simulink model "mbdt_autosar_system_top"  (R2019a)
settings: Solver=ode4  StartTime=0  StopTime=1.5  FixedStep=0.005  RelTol=1e-3  EnableMultiTasking=on
InitFcn:
  | mbd_s32k_as_consistency_checks(bdroot(gcs));
model workspace (MAT data in the model file):
  HBridgeCmd_LkupTbl = Simulink.LookupTable
  HBridgeCmd_LkupTbl.Table = Simulink.lookuptable.Table
  HBridgeCmd_LkupTbl.Table.Value = [-2048 -1843 -1638 -1434 -1229 -1024 -819 -614 -410 -205 0 205 410 614 819 1024 1229 1434 1638 1843 2048]
  HBridgeCmd_LkupTbl.Table.Dimensions = [1 21]
  HBridgeCmd_LkupTbl.Table.DataType = 'int16'
  HBridgeCmd_LkupTbl.Table.FieldName = 'Table'
  HBridgeCmd_LkupTbl.Breakpoints = Simulink.lookuptable.Breakpoint
  HBridgeCmd_LkupTbl.Breakpoints.Value = [-100 -90 -80 -70 -60 -50 -40 -30 -20 -10 0 10 20 30 40 50 60 70 80 90 100]
  HBridgeCmd_LkupTbl.Breakpoints.TunableSizeName = 'N1'
  HBridgeCmd_LkupTbl.Breakpoints.Dimensions = [1 21]
  HBridgeCmd_LkupTbl.Breakpoints.DataType = 'single'
  HBridgeCmd_LkupTbl.Breakpoints.FieldName = 'BP1'
  HBridgeCmd_LkupTbl.SupportTunableSize = 0
  HBridgeCmd_LkupTbl.StructTypeInfo = Simulink.lookuptable.StructTypeInfo
  HBridgeCmd_LkupTbl.StructTypeInfo.Name = 'MyStruct_Actuator'
  HBridgeCmd_LkupTbl.StructTypeInfo.DataScope = 'Auto'
  J = 0.226199211484
  Kt = 174.53
  SetpointPercent_LkupTbl = Simulink.LookupTable
  SetpointPercent_LkupTbl.Table = Simulink.lookuptable.Table
  SetpointPercent_LkupTbl.Table.Value = [0 10 20 30 40 50 60 70 80 90 100]
  SetpointPercent_LkupTbl.Table.Dimensions = [1 11]
  SetpointPercent_LkupTbl.Table.DataType = 'single'
  SetpointPercent_LkupTbl.Table.FieldName = 'Table'
  SetpointPercent_LkupTbl.Breakpoints = Simulink.lookuptable.Breakpoint
  SetpointPercent_LkupTbl.Breakpoints.Value = [170 251.5 333 414.5 496 577.5 659 740.5 822 903.5 985]
  SetpointPercent_LkupTbl.Breakpoints.TunableSizeName = 'N1'
  SetpointPercent_LkupTbl.Breakpoints.Dimensions = [1 11]
  SetpointPercent_LkupTbl.Breakpoints.DataType = 'single'
  SetpointPercent_LkupTbl.Breakpoints.FieldName = 'BP1'
  SetpointPercent_LkupTbl.SupportTunableSize = 0
  SetpointPercent_LkupTbl.StructTypeInfo = Simulink.lookuptable.StructTypeInfo
  SetpointPercent_LkupTbl.StructTypeInfo.Name = 'MyStruct'
  SetpointPercent_LkupTbl.StructTypeInfo.DataScope = 'Auto'
  TPSPrimaryPercent_LkupTbl = Simulink.LookupTable
  TPSPrimaryPercent_LkupTbl.Table = Simulink.lookuptable.Table
  TPSPrimaryPercent_LkupTbl.Table.Value = [0 10 20 30 40 50 60 70 80 90 100]
  TPSPrimaryPercent_LkupTbl.Table.Dimensions = [1 11]
  TPSPrimaryPercent_LkupTbl.Table.DataType = 'single'
  TPSPrimaryPercent_LkupTbl.Table.FieldName = 'Table'
  TPSPrimaryPercent_LkupTbl.Breakpoints = Simulink.lookuptable.Breakpoint
  TPSPrimaryPercent_LkupTbl.Breakpoints.Value = [170 249.600006104 329.200012207 408.799987793 488.399993896 568 647.599975586 727.200012207 806.799987793 886.400024414 966]
  TPSPrimaryPercent_LkupTbl.Breakpoints.TunableSizeName = 'N1'
  TPSPrimaryPercent_LkupTbl.Breakpoints.Dimensions = [1 11]
  TPSPrimaryPercent_LkupTbl.Breakpoints.DataType = 'single'
  TPSPrimaryPercent_LkupTbl.Breakpoints.FieldName = 'BP1'
  TPSPrimaryPercent_LkupTbl.SupportTunableSize = 0
  TPSPrimaryPercent_LkupTbl.StructTypeInfo = Simulink.lookuptable.StructTypeInfo
  TPSPrimaryPercent_LkupTbl.StructTypeInfo.Name = 'MyStruct'
  TPSPrimaryPercent_LkupTbl.StructTypeInfo.DataScope = 'Auto'
  TPSSecondaryPercent_LkupTbl = Simulink.LookupTable
  TPSSecondaryPercent_LkupTbl.Table = Simulink.lookuptable.Table
  TPSSecondaryPercent_LkupTbl.Table.Value = [100 90 80 70 60 50 40 30 20 10 0]
  TPSSecondaryPercent_LkupTbl.Table.Dimensions = [1 11]
  TPSSecondaryPercent_LkupTbl.Table.DataType = 'single'
  TPSSecondaryPercent_LkupTbl.Table.FieldName = 'Table'
  TPSSecondaryPercent_LkupTbl.Breakpoints = Simulink.lookuptable.Breakpoint
  TPSSecondaryPercent_LkupTbl.Breakpoints.Value = [170 249.600006104 329.200012207 408.799987793 488.399993896 568 647.599975586 727.200012207 806.799987793 886.400024414 966]
  TPSSecondaryPercent_LkupTbl.Breakpoints.TunableSizeName = 'N1'
  TPSSecondaryPercent_LkupTbl.Breakpoints.Dimensions = [1 11]
  TPSSecondaryPercent_LkupTbl.Breakpoints.DataType = 'single'
  TPSSecondaryPercent_LkupTbl.Breakpoints.FieldName = 'BP1'
  TPSSecondaryPercent_LkupTbl.SupportTunableSize = 0
  TPSSecondaryPercent_LkupTbl.StructTypeInfo = Simulink.lookuptable.StructTypeInfo
  TPSSecondaryPercent_LkupTbl.StructTypeInfo.Name = 'MyStruct'
  TPSSecondaryPercent_LkupTbl.StructTypeInfo.DataScope = 'Auto'
  Ts_verif = Simulink.Parameter
  Ts_verif.Value = 0.001
  Ts_verif.DataType = 'auto'
  Ts_verif.Dimensions = [1 1]
  angle_init = 15
  angle_open = 85
  c = 8.89069171842
  dirtyFlag = 'off'
  fall_end_angle = Simulink.Parameter
  fall_end_angle.Value = 0.1
  fall_end_angle.DataType = 'auto'
  fall_end_angle.Dimensions = [1 1]
  fall_start_angle = Simulink.Parameter
  fall_start_angle.Value = 0.9
  fall_start_angle.DataType = 'auto'
  fall_start_angle.Dimensions = [1 1]
  input_delay = 0.00986306560803
  k = 19.1559540807
  rise_end_angle = Simulink.Parameter
  rise_end_angle.Value = 0.9
  rise_end_angle.DataType = 'auto'
  rise_end_angle.Dimensions = [1 1]
  rise_start_angle = Simulink.Parameter
  rise_start_angle.Value = 0.1
  rise_start_angle.DataType = 'auto'
  rise_start_angle.Dimensions = [1 1]
  vv_fall_time_max = Simulink.Parameter
  vv_fall_time_max.Value = 0.3
  vv_fall_time_max.DataType = 'auto'
  vv_fall_time_max.Dimensions = [1 1]
  vv_fall_time_min = Simulink.Parameter
  vv_fall_time_min.Value = 0.001
  vv_fall_time_min.DataType = 'auto'
  vv_fall_time_min.Dimensions = [1 1]
  vv_rise_time_max = Simulink.Parameter
  vv_rise_time_max.Value = 0.1
  vv_rise_time_max.DataType = 'auto'
  vv_rise_time_max.Dimensions = [1 1]
  vv_rise_time_min = Simulink.Parameter
  vv_rise_time_min.Value = 0.001
  vv_rise_time_min.DataType = 'auto'
  vv_rise_time_min.Dimensions = [1 1]
undefined symbols (not defined in the file or in its folder): sigbuilder_block
libraries: simulink x1
Description:
  | This model shows how to run a throttle position control system AUTOSAR simulation in PIL mode on S32K targets.
  | The model is based on the Matlab's AUTOSAR Blockset Toolbox  'autosar_composition' example. The initial model is a composition containing six interconnected AUTOSAR software components.
  | More details about it can be found here https://www.mathworks.com/help/autosar/ug/example-design-autosar-components.html.
  | 
  | In order to run the entire simulation on S32K target in PIL mode, all the model components were unified in the mbdt_autosar_system.slx model. This was refferenced in the mbdt_autosar_system_top.slx model and
  | the mbdt_autosar_system will be run on target.
  | 
  | In order to run this model in PIL simulation on target, the following steps must be followed:
  | 1. Open the reference 'mbdt_autosar_system' model.
  | 2. Open the 'MBD_S32K1xx_AUTOSAR_Config_Information' block. If you want to run a custom/another AUTOSAR compliant model in PIL, once it runs in simulation as expected, this block must be added in the model.
  | It will change the System target file and will perform the model settings for code build and target deployment.
  | 3. In the MCU Tab chose the processor on which you want to run the model. For S32K11x EVB, the Clock and XTAL Frequency must be 40 MHz/External 40MHz. For the other boards the frequencies must be chosen
  | 80/External 8 MHz.
  | 4. In Build Toolchain Tab select the Compiler which you want to use.
  | 5. In Target Connection Tab Select the Download Interface type: Serial/OpenSDA. The Serial Group selects the computer COM port on which the Matlab model will exchange data with the target and the desired Baud Rate.
  | The OpenSDA group will be active only if the Download Interface is OpenSDA. Here, the right EVB Drive Name must be selected.
  | The PIL Settings Tab selects the EVB board LPUART instance and pins used for the PIL Serial communication. For the S32K11x must be selected the LPUART0/PTB0/PTB1 configuration. For the S32K14x must be selected
  | the LPUART1/PTC6/PTC7 configuration.
  | 6. Save the model and return to the top model.
  | 7. If the top model was never been run on the S32K board, go tho Tools>NXP Model-Based Design AUTOSAR Toolbox for  S32K1xx MCUs>To PIL Mode on S32K.
  | 8. Press Run button.
  | The code will be generated, compiledd, deployed and run on the target.
settings Model: OrderedModelArguments=off  Creator=NXP MBDT Team  LastModifiedBy=nxf35401
settings DataIOCC: SaveFormat=Array  SaveOutput=off  SaveTime=off  ReturnWorkspaceOutputs=off  SignalLoggingName=DataLog
settings OptimizationCC: BooleanDataType=off  DefaultParameterBehavior=Inlined  InlineInvariantSignals=on  EnhancedBackFolding=on  PassReuseOutputArgsAs=Individual arguments  ExpressionDepthLimit=2147483647  ZeroExternalMemoryAtStartup=off  ZeroInternalMemoryAtStartup=off  InitFltsAndDblsToZero=on  NoFixptDivByZeroProtection=on  EfficientFloat2IntCast=on  BufferReusableBoundary=off  OptimizeBlockOrder=speed  DifferentSizesBufferReuse=on
settings DebuggingCC: SaveWithParameterizedLinksMsg=none  MultiTaskDSMMsg=warning  IntegerOverflowMsg=none  ParameterTunabilityLossMsg=error  FcnCallInpInsideContextMsg=warning  BusObjectLabelMismatch=none  StateNameClashWarn=warning  SFUnexpectedBacktrackingDiag=warning  SFNoUnconditionalDefaultTransitionDiag=warning  SFExecutionAtInitializationDiag=none  ArithmeticOperatorsInVariantConditions=warning
settings HardwareCC: ProdBitPerPointer=32  ProdBitPerSizeT=32  ProdBitPerPtrDiffT=32  ProdLargestAtomicInteger=Long  ProdLargestAtomicFloat=Double  ProdWordSize=32  ProdHWDeviceType=ARM Compatible->ARM Cortex
settings ModelReferenceCC: PropagateSignalLabelsOutOfModel=off
settings SFSimCC: SimUseLocalCustomCode=off  SimParseCustomCode=off  MATLABDynamicMemAlloc=off
settings RTWCC: SystemTargetFile=mbd_s32k_as.tlc  MakeCommand=mbd_s32k_as_make_rtw COPY_MDLREF_INCLUDES=0  TemplateMakefile=mbd_s32k_as.tmf  Description=Model Based Design Autosar Toolbox S32K Code Generation Target  GenerateReport=on  RTWUseLocalCustomCode=off  IncludeHyperlinkInReport=on  LaunchReport=on  CodeExecutionProfiling=on  CodeProfilingInstrumentation=detailed  GenerateTraceInfo=on  GenerateTraceReport=on  GenerateTraceReportSl=on  GenerateTraceReportSf=on  GenerateTraceReportEml=on
settings CodeAppCC: ForceParamTrailComments=on  IgnoreCustomStorageClasses=off  MaxIdLength=63  OperatorAnnotations=on  SimulinkDataObjDesc=on  SFDataObjDesc=on  CustomSymbolStrType=$N$R$M  InsertBlockDesc=on  InternalIdentifier=Classic  ReqsInCode=on
settings STFCustomTargetCC: TargetLangStandard=C99 (ISO)  MultiwordLength=256  ParMdlRefBuildCompliant=on  CompOptLevelCompliant=on  IncludeMdlTerminateFcn=off  CombineOutputUpdateFcns=on  SuppressErrorStatus=on  ERTCustomFileBanners=on  SupportAbsoluteTime=off  MultiInstanceERTCode=on  CodeInterfacePackaging=Reusable function  SupportNonFinite=off  SupportComplex=off  SupportContinuousTime=off  SupportNonInlinedSFcns=off  RemoveResetFunc=on  MATLABClassNameForMDSCustomization=Simulink.SoftwareTarget.ERTCustomization  AutosarCompliant=on  GRTInterface=off  LookupTableObjectStructAxisOrder=2,1,3,4,...  LUTObjectStructOrderEvenSpacing=Size,Table,Breakpoints  SystemTargetFile=mbd_s32k_as.tlc
settings ERTTargetCC: TargetLangStandard=C99 (ISO)  ConcurrentExecutionCompliant=off  IncludeMdlTerminateFcn=off  SuppressErrorStatus=on  SupportAbsoluteTime=off  MultiInstanceERTCode=on  CodeInterfacePackaging=Reusable function  SupportNonFinite=off  SupportComplex=off  ModelStepFunctionPrototypeControlCompliant=off  CPPClassGenCompliant=off  AutosarCompliant=on  UseToolchainInfoCompliant=off  LookupTableObjectStructAxisOrder=2,1,3,4,...  LUTObjectStructOrderEvenSpacing=Size,Table,Breakpoints  InlinedParameterPlacement=NonHierarchical  ERTCustomFileTemplate=example_file_process.tlc
settings ConfigComp: CovMetricSettings=dw  CovHtmlReporting=on  CovSaveCumulativeToWorkspaceVar=on  CovSaveSingleToWorkspaceVar=on  CovExternalEMLEnable=off
settings SimscapeCC: SimscapeNormalizeSystem=off

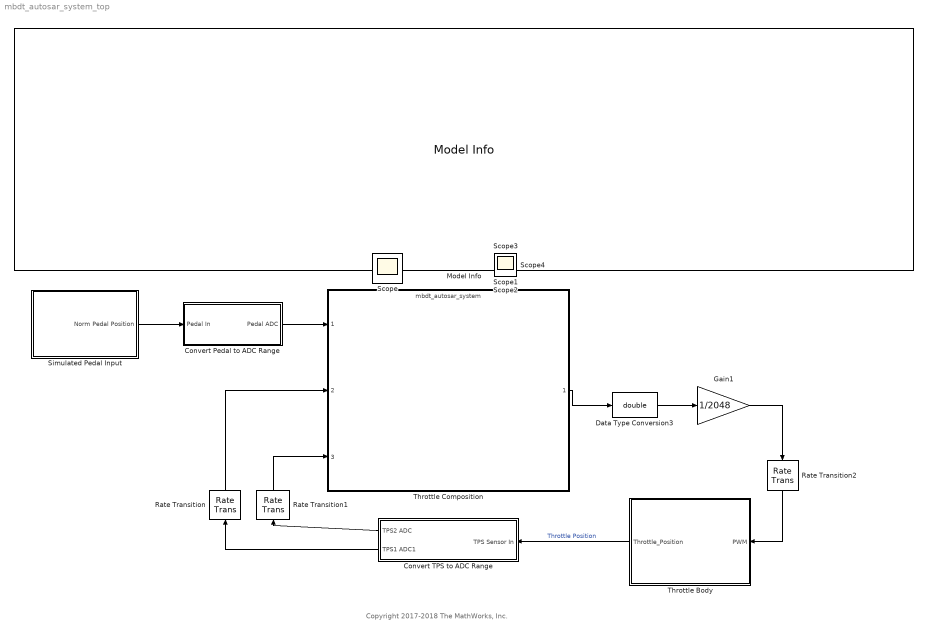
== system mbdt_autosar_system_top ==
  note: Copyright 2017-2018 The MathWorks, Inc.
  Convert Pedal to ADC Range : Subsystem
  Convert TPS to ADC Range : Subsystem
  Data Type Conversion3 : DataTypeConversion  OutDataTypeStr=double
  Gain1 : Gain  Gain=1/2048
  Model Info : simulink/Model-Wide Utilities/Model Info  Frame=off  DisplayStringWithTags=|  HorizontalTextAlignment=Left  LeftAlignmentValue=0.02
      | Model Name: %<ModelName>
      | 
      | Description: %<Description>
  Rate Transition : RateTransition  Deterministic=off  OutPortSampleTime=.005
  Rate Transition1 : RateTransition  Deterministic=off  OutPortSampleTime=.005
  Rate Transition2 : RateTransition  Deterministic=off
  Simulated Pedal Input : Subsystem  mask{groupIndex=WOT Pulse}
      mask prompts: groupIndex "Select Signal Group"
      mask help:
      | To use this block in a Simulink model, add the following code to the model
      | InitFcn callback:
      | groupIndex = get_param([gcs,'/Simulated Pedal Input'], 'MaskWSVariables');
      | signalbuilder([gcs,'/Simulated Pedal Input/Test Signals'], 'activegroup', groupIndex.Value);
      mask TypeOptions groupIndex: WOT Step | WOT Pulse | 60% Pulse | Sinusoidal Pulsetrain
      mask Display: image('pedal.jpg')
  Throttle Body : Subsystem  mask{units=normalized, input_delay=input_delay, J=J, c=c, k=k, close_angle=angle_init, open_angle=angle_open}
      mask prompts: input_delay "Input Delay:"; J "Inertia:"; c "Damping:"; k "Stiffness:"; close_angle "Resting Angle:"; open_angle "Open Angle:"
      mask TypeOptions units: rads | degrees | normalized
      mask Display: image('throttle.jpg')
  Throttle Composition : ModelReference  ModelNameDialog=mbdt_autosar_system.slx  SimulationMode=Processor-in-the-loop (PIL)  CachedPortDiscreteRates=[0.005]  CodeInterface=Top model  ModelReferenceVersion=1.71
  Scope{,1..4} (5 alike) : Scope
  wires:
  Throttle Composition/1 -> Data Type Conversion3/1
  Convert TPS to ADC Range/2(TPS1 ADC1) -> Rate Transition/1
  Gain1/1 -> Rate Transition2/1
  Data Type Conversion3/1 -> Gain1/1
  Convert TPS to ADC Range/1(TPS2 ADC) -> Rate Transition1/1
  Throttle Body/1(Throttle_Position) -> Convert TPS to ADC Range/1(TPS Sensor In)  "Throttle Position"
  Simulated Pedal Input/1(Norm Pedal Position) -> Convert Pedal to ADC Range/1(Pedal In)
  Convert Pedal to ADC Range/1(Pedal ADC) -> Throttle Composition/1
  Rate Transition2/1 -> Throttle Body/1(PWM)
  Rate Transition/1 -> Throttle Composition/2
  Rate Transition1/1 -> Throttle Composition/3

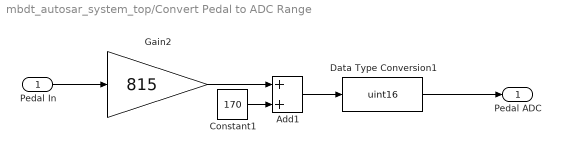
== system mbdt_autosar_system_top/Convert Pedal to ADC Range ==
  Pedal In : Inport
  Add1 : Sum
  Constant1 : Constant  Value=170
  Data Type Conversion1 : DataTypeConversion  OutDataTypeStr=uint16
  Gain2 : Gain  Gain=815
  Pedal ADC : Outport
  wires:
  Gain2/1 -> Add1/1
  Constant1/1 -> Add1/2
  Data Type Conversion1/1 -> Pedal ADC/1
  Add1/1 -> Data Type Conversion1/1
  Pedal In/1 -> Gain2/1

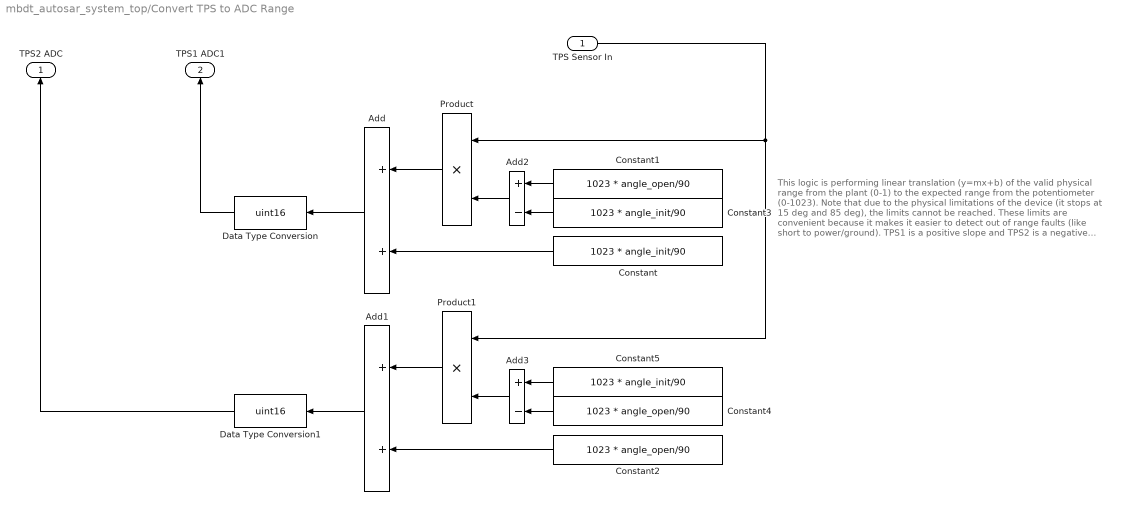
== system mbdt_autosar_system_top/Convert TPS to ADC Range ==
  note: This logic is performing linear translation (y=mx+b) of the valid physical range from the plant (0-1) to the expected range from the potentiometer (0-1023).
      |
      | Note that due to the physical limitations of the device (it stops at 15 deg and 85 deg), the limits cannot be reached.
      |
      | These limits are convenient because it makes it easier to detect out of range faults (like short to power/ground).
      |
      | TPS1 is a positive slope and TPS2 is a negative slope.  This is common in these devices so cross checking between the two sensors can be performed.
  TPS Sensor In : Inport
  Add : Sum
  Add1 : Sum
  Add2 : Sum  Inputs=+-
  Add3 : Sum  Inputs=+-
  Constant : Constant  Value=1023 * angle_init/90
  Constant1 : Constant  Value=1023 * angle_open/90
  Constant2 : Constant  Value=1023 * angle_open/90
  Constant3 : Constant  Value=1023 * angle_init/90
  Constant4 : Constant  Value=1023 * angle_open/90
  Constant5 : Constant  Value=1023 * angle_init/90
  Data Type Conversion : DataTypeConversion  OutDataTypeStr=uint16
  Data Type Conversion1 : DataTypeConversion  OutDataTypeStr=uint16
  Product : Product
  Product1 : Product
  TPS2 ADC : Outport
  TPS1 ADC1 : Outport  Port=2
  wires:
  Product/1 -> Add/1
  Constant/1 -> Add/2
  Add/1 -> Data Type Conversion/1
  Data Type Conversion/1 -> TPS1 ADC1/1
  Add1/1 -> Data Type Conversion1/1
  Add2/1 -> Product/2
  Constant1/1 -> Add2/1
  Constant3/1 -> Add2/2
  Constant4/1 -> Add3/2
  Constant5/1 -> Add3/1
  Add3/1 -> Product1/2
  Constant2/1 -> Add1/2
  Product1/1 -> Add1/1
  Data Type Conversion1/1 -> TPS2 ADC/1
  TPS Sensor In/1 -> Product1/1, Product/1

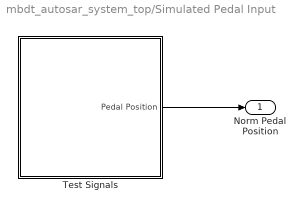
== system mbdt_autosar_system_top/Simulated Pedal Input ==
  Test Signals : Subsystem  Tag=STV Subsys  LoadFcn=sigbuilder_block('load');  StartFcn=sigbuilder_block('start');  StopFcn=sigbuilder_block('stop');  ClipboardFcn=sigbuilder_block('clipboard');  mask(Sigbuilder block){tuvar=[0:10]}
      mask help: Sigbuilder GUI
      mask init:
      | tuvar = sigbuilder_block('maskInit');
      settings: CopyFcn=sigbuilder_block('copy');  DeleteFcn=sigbuilder_block('delete');  ModelCloseFcn=sigbuilder_block('modelClose');  PreSaveFcn=sigbuilder_block('preSave');  PauseFcn=sigbuilder_block('pause')  ContinueFcn=sigbuilder_block('continue')  NameChangeFcn=sigbuilder_block('namechange');  OpenFcn=sigbuilder_block('open',[-1004.25 112.5 630 289.5 ]);  CloseFcn=sigbuilder_block('close');
      mask Display: plot(0, 0, 100, 100,[2, 2, 32, 32, 2], [68, 8, 8, 68, 68],[32, 2], [38, 38], [32, 19, 2],[53, 60, 44], [32, 17, 17, 2],[16, 16, 31, 31]);txt = getActiveGroup(gcbh);text(2, 100, txt,'verticalAlignment', 'top');
  Norm Pedal Position : Outport
  wires:
  Test Signals/1(Pedal Position) -> Norm Pedal Position/1

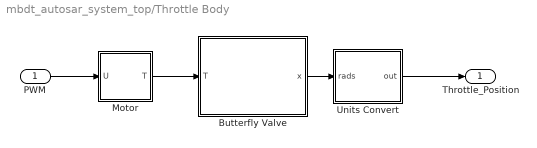
== system mbdt_autosar_system_top/Throttle Body ==
  PWM : Inport
  Butterfly Valve : Subsystem  mask{var_J=J, var_D=c, var_K=k, angle_init=angle_init, angle_open=angle_open}
      mask prompts: var_J "Inertia:"; var_D "Damping:"; var_K "Stiffness:"; angle_init "Resting Angle:"; angle_open "Open Angle:"
  Motor : Subsystem
  Units Convert : Subsystem
  Throttle_Position : Outport
  wires:
  PWM/1 -> Motor/1(U)
  Motor/1(T) -> Butterfly Valve/1(T)
  Units Convert/1(out) -> Throttle_Position/1
  Butterfly Valve/1(x) -> Units Convert/1(rads)

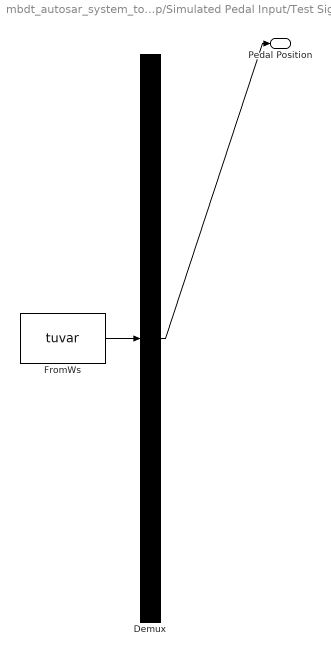
== system mbdt_autosar_system_top/Simulated Pedal Input/Test Signals ==
  Demux : Demux  Tag=STV Demux  Outputs=1
  FromWs : FromWorkspace  Tag=STV FromWs  VariableName=tuvar  SampleTime=0
      SigBuilderData=|
      | dataSet(1).timeRange = [0 1.5]
      | dataSet(1).name = 'WOT Step'
      | dataSet(2).timeRange = [0 1.5]
      | dataSet(2).name = 'WOT Pulse'
      | dataSet(3).timeRange = [0 1.5]
      | dataSet(3).name = '60% Pulse'
      | dataSet(4).timeRange = [0 10]
      | dataSet(4).name = 'Pulse'
      | sbobj.Groups(1).Name = 'WOT Step'
      | sbobj.Groups(1).Signals.Name = 'Pedal Position'
      | sbobj.Groups(1).Signals.XData = [0 0.05 0.05 0.101 1 1.5]
      | sbobj.Groups(1).Signals.YData = [0 0 1 1 1 1]
      | sbobj.Groups(1).TimeRange = [0 1.5]
      | sbobj.Groups(2).Name = 'WOT Pulse'
      | sbobj.Groups(2).Signals.Name = 'Pedal Position'
      | sbobj.Groups(2).Signals.XData = [0 0.05 0.05 0.101 1 1 1.5]
      | sbobj.Groups(2).Signals.YData = [0 0 1 1 1 0 0]
      | sbobj.Groups(2).TimeRange = [0 1.5]
      | sbobj.Groups(3).Name = '60% Pulse'
      | sbobj.Groups(3).Signals.Name = 'Pedal Position'
      | sbobj.Groups(3).Signals.XData = [0 0.05 0.05 1 1 1.5]
      | sbobj.Groups(3).Signals.YData = [0 0 0.6 0.6 0 0]
      | sbobj.Groups(3).TimeRange = [0 1.5]
      | sbobj.Groups(4).Name = 'Pulse'
      | sbobj.Groups(4).Signals.Name = 'Pedal Position'
      | sbobj.Groups(4).Signals.XData = [0 0.1 0.2 0.3 0.4 0.5 0.6 0.7 0.8 0.9 1 1 1.1 1.2 1.3 1.4 1.5 1.6 1.7 1.8 1.9 2 2 2.1 2.2 2.3 2.4 2.5 2.6 2.7 2.8 2.9 3 3 3.1 3.2 3.3 3.4 3.5 3.6 3.7 3.8 3.9 4 4 4.1 4.2 4.3 4.4 4.5 4.6 4.7 4.8 4.9 5 5 5.1 5.2 5.3 5.4 5.5 5.6 5.7 5.8 5.9 6 6 6.1 6.2 6.3 6.4 6.5 6.6 6.7 6.8 6.9 7 7 7.1 7.2 7.3 7.4 7.5 7.6 7.7 7.8 7.9 8 8 8.1 8.2 8.3 8.4 8.5 8.6 8.7 8.8 8.9 9 9 9.1 9.2 9.3 9.4 9.5 9.6 9.7 9.8 9.9 10]
      | sbobj.Groups(4).Signals.YData = [0.5 0.793892626146 0.975528258148 0.975528258148 0.793892626146 0.5 0.206107373854 0.0244717418524 0.0244717418524 0.206107373854 0.5 0.5 0.793892626146 0.975528258148 0.975528258148 0.793892626146 0.5 0.206107373854 0.0244717418524 0.0244717418524 0.206107373854 0.5 0.5 0.793892626146 0.975528258148 0.975528258148 0.793892626146 0.5 0.206107373854 0.0244717418524 0.0244717418524 0.206107373854 0.5 0.5 0.793892626146 0.975528258148 0.975528258148 0.793892626146 0.5 0.206107373854 0.0244717418524 0.0244717418524 0.206107373854 0.5 0.5 0.793892626146 0.975528258148 0.975528258148 0.793892626146 0.5 0.206107373854 0.0244717418524 0.0244717418524 0.206107373854 0.5 0.5 0.793892626146 0.975528258148 0.975528258148 0.793892626146 0.5 0.206107373854 0.0244717418524 0.0244717418524 0.206107373854 0.5 0.5 0.793892626146 0.975528258148 0.975528258148 0.793892626146 0.5 0.206107373854 0.0244717418524 0.0244717418524 0.206107373854 0.5 0.5 0.793892626146 0.975528258148 0.975528258148 0.793892626146 0.5 0.206107373854 0.0244717418524 0.0244717418524 0.206107373854 0.5 0.5 0.793892626146 0.975528258148 0.975528258148 0.793892626146 0.5 0.206107373854 0.0244717418524 0.0244717418524 0.206107373854 0.5 0.5 0.793892626146 0.975528258148 0.975528258148 0.793892626146 0.5 0.206107373854 0.0244717418524 0.0244717418524 0.206107373854 0.5]
  Pedal Position : Outport  Tag=STV Outport
  wires:
  Demux/1 -> Pedal Position/1
  FromWs/1 -> Demux/1

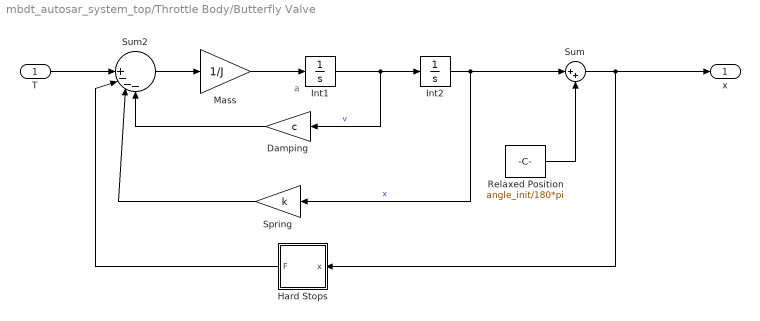
== system mbdt_autosar_system_top/Throttle Body/Butterfly Valve ==
  note: a
  T : Inport
  Damping : Gain  Gain=c  SaturateOnIntegerOverflow=on  OutDataTypeStr=Inherit: Same as input  ParamDataTypeStr=Inherit: Same as input
  Hard Stops : Subsystem  mask{H=angle_open/180*pi, K=2.86e5, L=angle_init/180*pi}
      mask prompts: H "Upper Limit:"; K "Stiffness:"; L "Lower Limit:"
  Int1 : Integrator
  Int2 : Integrator
  Mass : Gain  Gain=1/J  SaturateOnIntegerOverflow=on  OutDataTypeStr=Inherit: Same as input  ParamDataTypeStr=Inherit: Same as input
  Relaxed Position : Constant  Value=angle_init/180*pi
  Spring : Gain  Gain=k  SaturateOnIntegerOverflow=on  OutDataTypeStr=Inherit: Same as input  ParamDataTypeStr=Inherit: Same as input
  Sum : Sum  Inputs=|++  SaturateOnIntegerOverflow=on  InputSameDT=on  OutDataTypeStr=Inherit: Same as first input
  Sum2 : Sum  Inputs=|||+---  SaturateOnIntegerOverflow=on  InputSameDT=on  OutDataTypeStr=Inherit: Same as first input
  x : Outport
  wires:
  Hard Stops/1(F) -> Sum2/2
  Spring/1 -> Sum2/3
  Int2/1 -> Spring/1, Sum/1  "x"
  Relaxed Position/1 -> Sum/2
  Sum2/1 -> Mass/1
  T/1 -> Sum2/1
  Mass/1 -> Int1/1
  Int1/1 -> Damping/1, Int2/1  "v"
  Damping/1 -> Sum2/4
  Sum/1 -> x/1, Hard Stops/1(x)

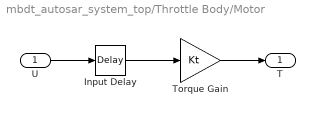
== system mbdt_autosar_system_top/Throttle Body/Motor ==
  U : Inport
  Input Delay : TransportDelay  DelayTime=input_delay
  Torque Gain : Gain  Gain=Kt  SaturateOnIntegerOverflow=on  OutDataTypeStr=Inherit: Same as input  ParamDataTypeStr=Inherit: Same as input
  T : Outport
  wires:
  U/1 -> Input Delay/1
  Torque Gain/1 -> T/1
  Input Delay/1 -> Torque Gain/1

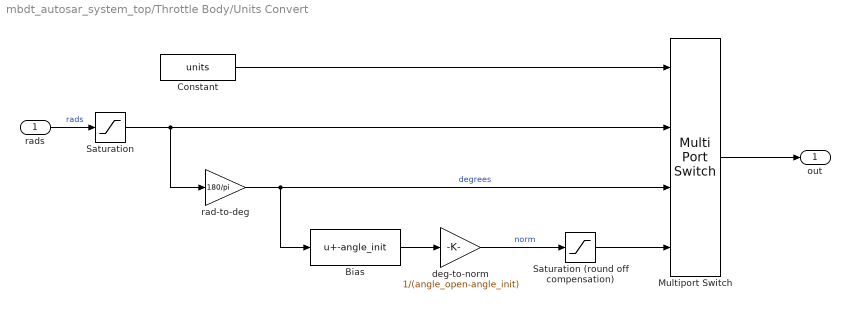
== system mbdt_autosar_system_top/Throttle Body/Units Convert ==
  rads : Inport
  Bias : Bias  Bias=-angle_init
  Constant : Constant  Value=units
  Multiport Switch : MultiPortSwitch
  Saturation : Saturate  UpperLimit=pi/2  LowerLimit=0.0
  Saturation (round off compensation) : Saturate  UpperLimit=1.0  LowerLimit=0.0
  deg-to-norm : Gain  Gain=1/(angle_open-angle_init)
      settings: AttributesFormatString=%<Gain>
  rad-to-deg : Gain  Gain=180/pi
  out : Outport
  wires:
  Saturation/1 -> rad-to-deg/1, Multiport Switch/2
  Saturation (round off compensation)/1 -> Multiport Switch/4
  Bias/1 -> deg-to-norm/1
  deg-to-norm/1 -> Saturation (round off compensation)/1  "norm"
  Constant/1 -> Multiport Switch/1
  Multiport Switch/1 -> out/1
  rads/1 -> Saturation/1  "rads"
  rad-to-deg/1 -> Multiport Switch/3, Bias/1  "degrees"

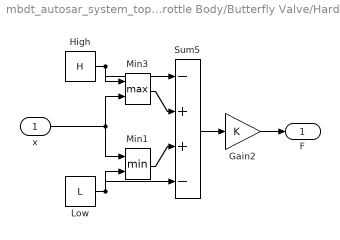
== system mbdt_autosar_system_top/Throttle Body/Butterfly Valve/Hard Stops ==
  x : Inport
  Gain2 : Gain  Gain=K  SaturateOnIntegerOverflow=on  OutDataTypeStr=Inherit: Same as input  ParamDataTypeStr=Inherit: Same as input
  High : Constant  Value=H
  Low : Constant  Value=L
  Min1 : MinMax  Inputs=2  SaturateOnIntegerOverflow=on  InputSameDT=on
  Min3 : MinMax  Function=max  Inputs=2  SaturateOnIntegerOverflow=on  InputSameDT=on
  Sum5 : Sum  Inputs=-+||+-  SaturateOnIntegerOverflow=on  InputSameDT=on  OutDataTypeStr=Inherit: Same as first input
  F : Outport
  wires:
  Gain2/1 -> F/1
  x/1 -> Min1/1, Min3/2
  Sum5/1 -> Gain2/1
  Low/1 -> Min1/2, Sum5/4
  High/1 -> Sum5/1, Min3/1
  Min3/1 -> Sum5/2
  Min1/1 -> Sum5/3
